simulink library "lib_Flight_Controller"  (R2019b)
settings: Solver=VariableStepAuto  StartTime=0.0  StopTime=10.0  RelTol=1e-3
undefined symbols (not defined in the file): FCC_PIX_Data, HIL_Data
settings Model: Creator=m.hiepp  LastModifiedBy=guy-m
settings DataIOCC: ReturnWorkspaceOutputs=off
settings DebuggingCC: ArithmeticOperatorsInVariantConditions=warning
settings SFSimCC: CustomCodeUndefinedFunction=UseInterfaceOnly

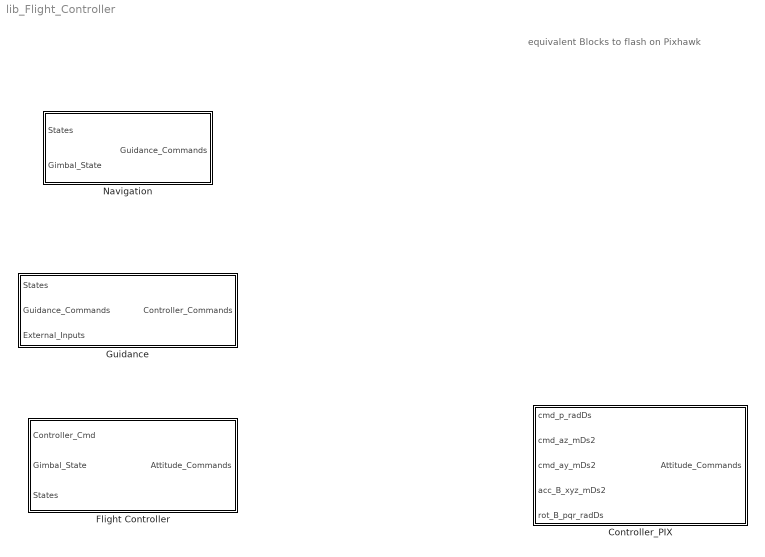
== system lib_Flight_Controller ==
  note: equivalent Blocks to flash on Pixhawk
  Controller_PIX : Subsystem
  Flight Controller : Subsystem  mask{FCC=HIL_Data.Flight_Controller}
      mask prompts: FCC "FCC Data"
  Guidance : Subsystem
  Navigation : Subsystem

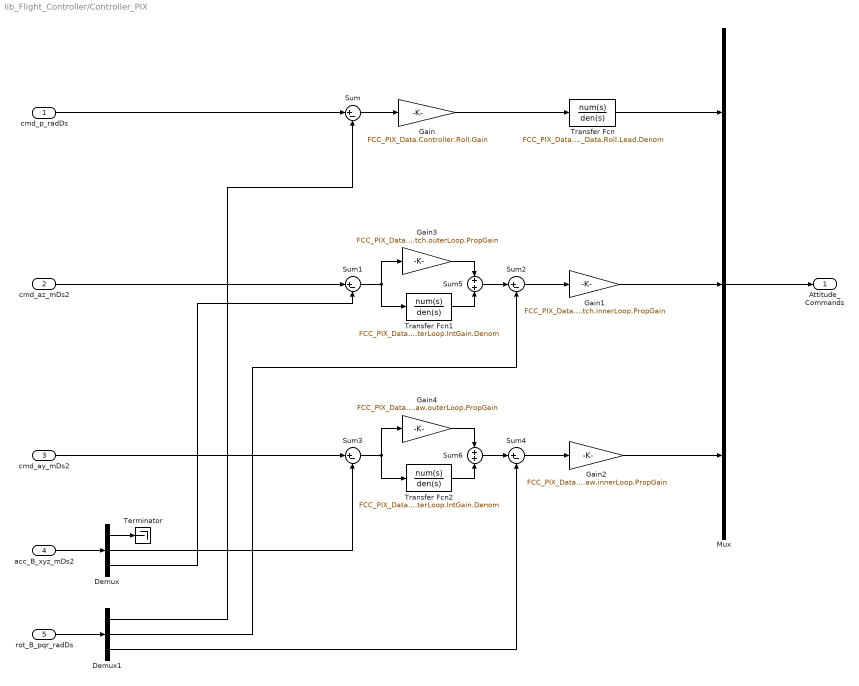
== system lib_Flight_Controller/Controller_PIX ==
  cmd_p_radDs : Inport
  cmd_az_mDs2 : Inport  Port=2
  cmd_ay_mDs2 : Inport  Port=3
  acc_B_xyz_mDs2 : Inport  Port=4
  rot_B_pqr_radDs : Inport  Port=5
  Demux : Demux  Outputs=3
  Demux1 : Demux  Outputs=3
  Gain : Gain  Gain=FCC_PIX_Data.Controller.Roll.Gain
  Gain1 : Gain  Gain=FCC_PIX_Data.Controller.Pitch.innerLoop.PropGain
  Gain2 : Gain  Gain=FCC_PIX_Data.Controller.Yaw.innerLoop.PropGain
  Gain3 : Gain  Gain=FCC_PIX_Data.Controller.Pitch.outerLoop.PropGain
  Gain4 : Gain  Gain=FCC_PIX_Data.Controller.Yaw.outerLoop.PropGain
  Mux : Mux  Inputs=3
  Sum{,1..4} (5 alike) : Sum  Inputs=|+-
  Sum5 : Sum  Inputs=+|+
  Sum6 : Sum  Inputs=+|+
  Terminator : Terminator
  Transfer Fcn : TransferFcn  Numerator=FCC_PIX_Data.Roll.Lead.Num  Denominator=FCC_PIX_Data.Roll.Lead.Denom
  Transfer Fcn1 : TransferFcn  Numerator=FCC_PIX_Data.Controller.Pitch.outerLoop.IntGain.Num  Denominator=FCC_PIX_Data.Controller.Pitch.outerLoop.IntGain.Denom
  Transfer Fcn2 : TransferFcn  Numerator=FCC_PIX_Data.Controller.Yaw.outerLoop.IntGain.Num  Denominator=FCC_PIX_Data.Controller.Yaw.outerLoop.IntGain.Denom
  Attitude_Commands : Outport  VectorParamsAs1DForOutWhenUnconnected=off
  wires:
  Sum6/1 -> Sum4/1
  Sum1/1 -> Transfer Fcn1/1, Gain3/1
  Gain3/1 -> Sum5/1
  Transfer Fcn1/1 -> Sum5/2
  Sum5/1 -> Sum2/1
  Gain/1 -> Transfer Fcn/1
  Sum2/1 -> Gain1/1
  Sum4/1 -> Gain2/1
  Sum/1 -> Gain/1
  Gain4/1 -> Sum6/1
  Transfer Fcn2/1 -> Sum6/2
  Sum3/1 -> Transfer Fcn2/1, Gain4/1
  cmd_p_radDs/1 -> Sum/1
  cmd_ay_mDs2/1 -> Sum3/1
  cmd_az_mDs2/1 -> Sum1/1
  Gain2/1 -> Mux/3
  Gain1/1 -> Mux/2
  Transfer Fcn/1 -> Mux/1
  Mux/1 -> Attitude_Commands/1
  acc_B_xyz_mDs2/1 -> Demux/1
  rot_B_pqr_radDs/1 -> Demux1/1
  Demux1/1 -> Sum/2
  Demux1/2 -> Sum2/2
  Demux1/3 -> Sum4/2
  Demux/2 -> Sum3/2
  Demux/3 -> Sum1/2
  Demux/1 -> Terminator/1

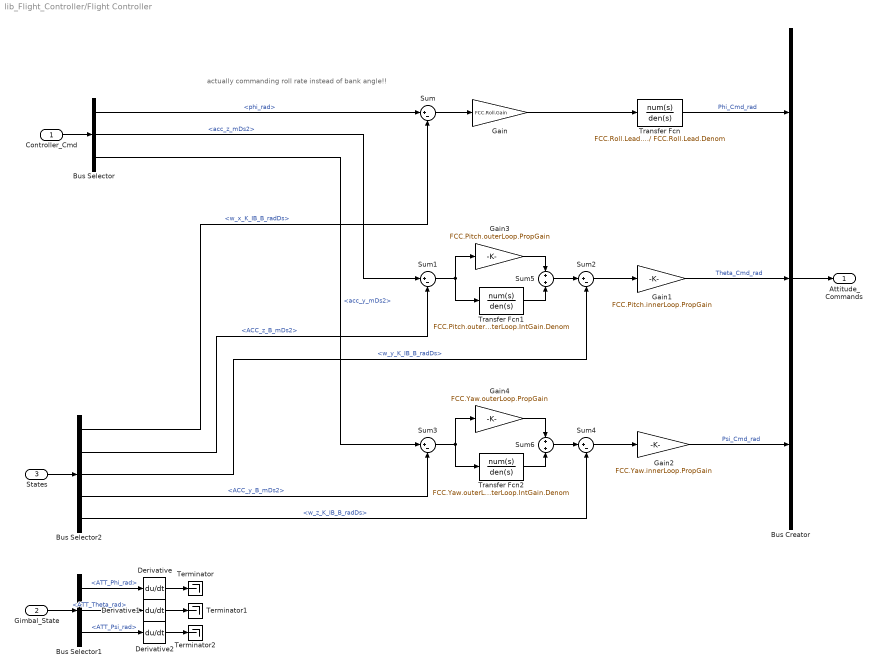
== system lib_Flight_Controller/Flight Controller ==
  note: actually commanding roll rate instead of bank angle!!
  Controller_Cmd : Inport  OutDataTypeStr=Bus: Controller_Cmd_Bus
  Gimbal_State : Inport  Port=2  OutDataTypeStr=Bus: Gimbal_State_Bus
  States : Inport  Port=3  OutDataTypeStr=Bus: States_Bus
  Bus Creator : BusCreator  Inputs=3  OutDataTypeStr=Bus: ATT_Cmd_Bus
  Bus Selector : BusSelector  OutputSignals=phi_rad,acc_z_mDs2,acc_y_mDs2
  Bus Selector1 : BusSelector  OutputSignals=Gimbal_Attitude.ATT_Euler.ATT_Phi_rad,Gimbal_Attitude.ATT_Euler.ATT_Theta_rad,Gimbal_Attitude.ATT_Euler.ATT_Psi_rad
  Bus Selector2 : BusSelector  OutputSignals=Rigid_Body_States.Rotation_States.w_x_K_IB_B_radDs,Rigid_Body_States.Acceleration_States.ACC_z_B_mDs2,Rigid_Body_States.Rotation_States.w_y_K_IB_B_radDs,Rigid_Body_States.Acceleration_States.ACC_y_B_mDs2,Rigid_Body_States.Rotation_States.w_z_K_IB_B_radDs
  Derivative : Derivative
  Derivative1 : Derivative
  Derivative2 : Derivative
  Gain : Gain  Gain=FCC.Roll.Gain
  Gain1 : Gain  Gain=FCC.Pitch.innerLoop.PropGain
  Gain2 : Gain  Gain=FCC.Yaw.innerLoop.PropGain
  Gain3 : Gain  Gain=FCC.Pitch.outerLoop.PropGain
  Gain4 : Gain  Gain=FCC.Yaw.outerLoop.PropGain
  Sum{,1..4} (5 alike) : Sum  Inputs=|+-
  Sum5 : Sum  Inputs=+|+
  Sum6 : Sum  Inputs=+|+
  Terminator : Terminator
  Terminator1 : Terminator
  Terminator2 : Terminator
  Transfer Fcn : TransferFcn  Numerator=FCC.Roll.Lead.Num  Denominator=FCC.Roll.Lead.Denom
  Transfer Fcn1 : TransferFcn  Numerator=FCC.Pitch.outerLoop.IntGain.Num  Denominator=FCC.Pitch.outerLoop.IntGain.Denom
  Transfer Fcn2 : TransferFcn  Numerator=FCC.Yaw.outerLoop.IntGain.Num  Denominator=FCC.Yaw.outerLoop.IntGain.Denom
  Attitude_Commands : Outport  OutDataTypeStr=Bus: ATT_Cmd_Bus  VectorParamsAs1DForOutWhenUnconnected=off
  wires:
  Controller_Cmd/1 -> Bus Selector/1
  Bus Creator/1 -> Attitude_Commands/1
  Gimbal_State/1 -> Bus Selector1/1
  States/1 -> Bus Selector2/1
  Gain/1 -> Transfer Fcn/1
  Bus Selector/1 -> Sum/1  "<phi_rad>"
  Sum/1 -> Gain/1
  Transfer Fcn/1 -> Bus Creator/1  "Phi_Cmd_rad"
  Bus Selector1/1 -> Derivative/1  "<ATT_Phi_rad>"
  Sum1/1 -> Transfer Fcn1/1, Gain3/1
  Sum5/1 -> Sum2/1
  Sum2/1 -> Gain1/1
  Gain1/1 -> Bus Creator/2  "Theta_Cmd_rad"
  Sum6/1 -> Sum4/1
  Sum4/1 -> Gain2/1
  Sum3/1 -> Transfer Fcn2/1, Gain4/1
  Gain2/1 -> Bus Creator/3  "Psi_Cmd_rad"
  Bus Selector/2 -> Sum1/1  "<acc_z_mDs2>"
  Bus Selector/3 -> Sum3/1  "<acc_y_mDs2>"
  Bus Selector1/3 -> Derivative2/1  "<ATT_Psi_rad>"
  Bus Selector1/2 -> Derivative1/1  "<ATT_Theta_rad>"
  Derivative/1 -> Terminator/1
  Derivative1/1 -> Terminator1/1
  Derivative2/1 -> Terminator2/1
  Transfer Fcn1/1 -> Sum5/2
  Gain3/1 -> Sum5/1
  Gain4/1 -> Sum6/1
  Transfer Fcn2/1 -> Sum6/2
  Bus Selector2/1 -> Sum/2  "<w_x_K_IB_B_radDs>"
  Bus Selector2/2 -> Sum1/2  "<ACC_z_B_mDs2>"
  Bus Selector2/3 -> Sum2/2  "<w_y_K_IB_B_radDs>"
  Bus Selector2/4 -> Sum3/2  "<ACC_y_B_mDs2>"
  Bus Selector2/5 -> Sum4/2  "<w_z_K_IB_B_radDs>"

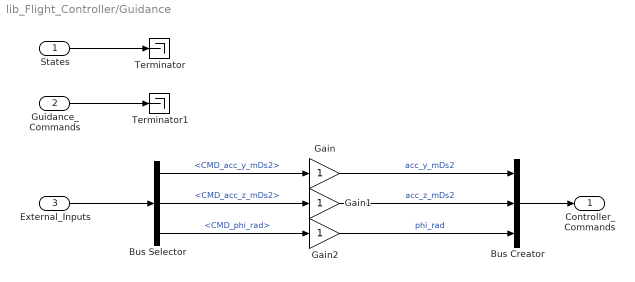
== system lib_Flight_Controller/Guidance ==
  States : Inport  OutDataTypeStr=Bus: States_Bus
  Guidance_Commands : Inport  Port=2  OutDataTypeStr=Bus: Guidance_Cmd_Bus
  External_Inputs : Inport  Port=3  OutDataTypeStr=Bus: External_Inputs_Bus
  Bus Creator : BusCreator  Inputs=3  OutDataTypeStr=Bus: Controller_Cmd_Bus
  Bus Selector : BusSelector  OutputSignals=FCC_External_Inputs.CMD_acc_y_mDs2,FCC_External_Inputs.CMD_acc_z_mDs2,FCC_External_Inputs.CMD_phi_rad
  Gain : Gain
  Gain1 : Gain
  Gain2 : Gain
  Terminator : Terminator
  Terminator1 : Terminator
  Controller_Commands : Outport  OutDataTypeStr=Bus: Controller_Cmd_Bus  VectorParamsAs1DForOutWhenUnconnected=off
  wires:
  Bus Creator/1 -> Controller_Commands/1
  External_Inputs/1 -> Bus Selector/1
  Bus Selector/1 -> Gain/1  "<CMD_acc_y_mDs2>"
  Bus Selector/2 -> Gain1/1  "<CMD_acc_z_mDs2>"
  Bus Selector/3 -> Gain2/1  "<CMD_phi_rad>"
  Guidance_Commands/1 -> Terminator1/1
  States/1 -> Terminator/1
  Gain/1 -> Bus Creator/1  "acc_y_mDs2"
  Gain2/1 -> Bus Creator/3  "phi_rad"
  Gain1/1 -> Bus Creator/2  "acc_z_mDs2"

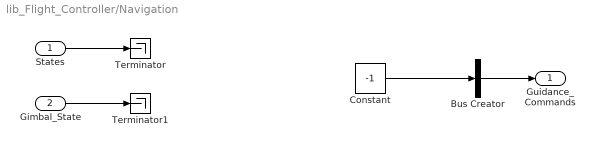
== system lib_Flight_Controller/Navigation ==
  States : Inport  OutDataTypeStr=Bus: States_Bus
  Gimbal_State : Inport  Port=2  OutDataTypeStr=Bus: Gimbal_State_Bus
  Bus Creator : BusCreator  Inputs=1  OutDataTypeStr=Bus: Guidance_Cmd_Bus
  Constant : Constant  Value=-1
  Terminator : Terminator
  Terminator1 : Terminator
  Guidance_Commands : Outport  OutDataTypeStr=Bus: Guidance_Cmd_Bus  VectorParamsAs1DForOutWhenUnconnected=off
  wires:
  Bus Creator/1 -> Guidance_Commands/1
  Constant/1 -> Bus Creator/1
  States/1 -> Terminator/1
  Gimbal_State/1 -> Terminator1/1
